simulink model "sampleModel1951"  (R2023a)
settings: Solver=VariableStepAuto  StartTime=0.0  StopTime=10.0  RelTol=1e-3
libraries: hdlsllib x3
settings Model: Creator=user1  LastModifiedBy=user1

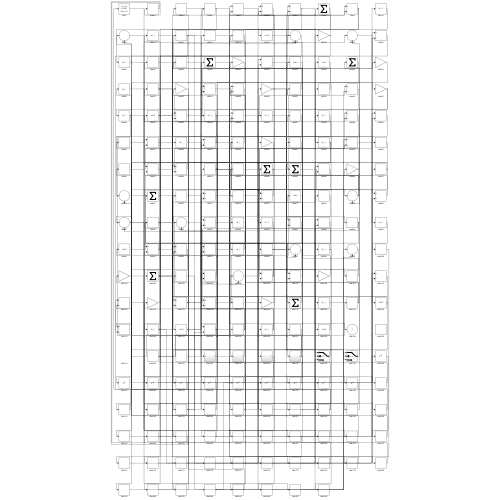
[thumbnail: Simulink's stored preview of the top-level diagram]
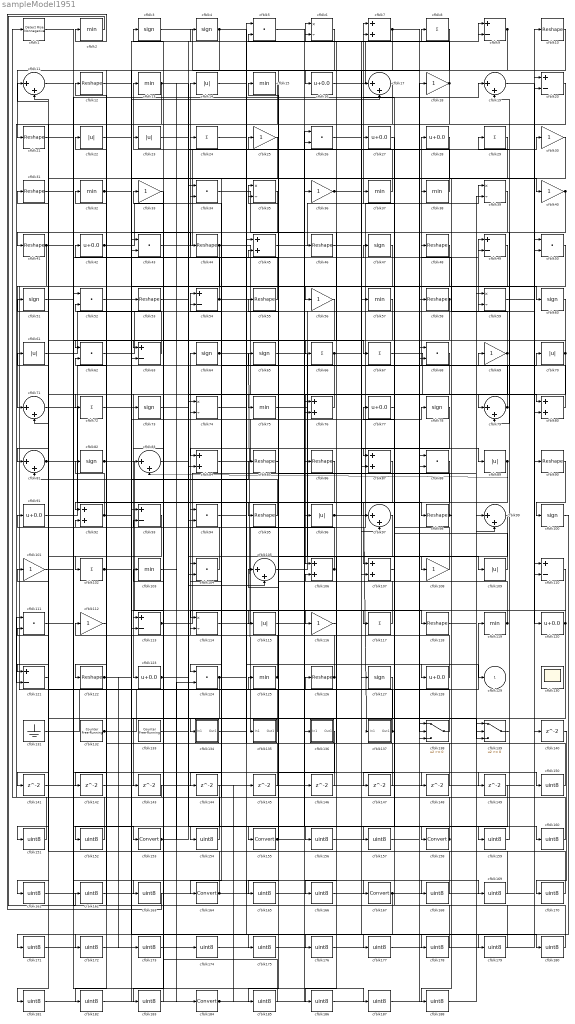
== system sampleModel1951 ==
  cfblk1 : hdlsllib/Logic and Bit Operations/Detect Rise Nonnegative  vinit=0  OutDataTypeStr=boolean
  cfblk{10,12,21,31,41,44,46,48,53,55,58,85..86,90,95,98,118,122,126} (19 alike) : Reshape
  cfblk{3..4,47,51,60,64..65,73,78,82,100,127} (12 alike) : Signum
  cfblk{18,25,30,33,36,40,56,69,101,108,112,116} (12 alike) : Gain
  cfblk{8,24,29,66..67,72,102,117} (8 alike) : Sum  Inputs=+
  cfblk{2,13,15,32,37..38,57,75,103,119,125} (11 alike) : MinMax
  cfblk{5,26,34,43,50,52,62,68,88,94,104,111,124} (13 alike) : DotProduct  OutDataTypeStr=Inherit: Inherit via internal rule
  cfblk{11,17,19,71,79,81,83,97,99,105} (10 alike) : Sum  Inputs=|++
  cfblk{7,45,76,80,84,87,92,106..107} (9 alike) : Sum
  cfblk{14,22..23,61,70,89,96,109,115} (9 alike) : Abs  SaturateOnIntegerOverflow=off
  cfblk{9,20,49,54,63,93,110,113,121} (9 alike) : Sum  Inputs=+-
  cfblk{6,35,39,59,74,114} (6 alike) : Product  Inputs=*/  RndMeth=Zero  SaturateOnIntegerOverflow=on
  cfblk{16,27..28,42,77,91,120,123,128} (9 alike) : Bias  Bias=0.0  SaturateOnIntegerOverflow=off
  cfblk130 : Scope
      settings: Floating=on
  cfblk131 : Ground
  cfblk132 : hdlsllib/Sources/Counter Free-Running  NumBits=16  tsamp=-1
  cfblk133 : hdlsllib/Sources/Counter Free-Running  NumBits=16  tsamp=-1
  cfblk134 : Subsystem
      settings: LibrarySourceBlock=|
      | hdlsllib/Ports &
      | Subsystems/Subsystem
  cfblk135 : Subsystem
      settings: LibrarySourceBlock=|
      | hdlsllib/Ports &
      | Subsystems/Subsystem
  cfblk136 : Subsystem
      settings: LibrarySourceBlock=|
      | hdlsllib/Ports &
      | Subsystems/Subsystem
  cfblk137 : Subsystem
      settings: LibrarySourceBlock=|
      | hdlsllib/Ports &
      | Subsystems/Subsystem
  cfblk138 : Switch  SaturateOnIntegerOverflow=off  InputSameDT=off
  cfblk139 : Switch  SaturateOnIntegerOverflow=off  InputSameDT=off
  cfblk{140..149} (10 alike) : Delay  SampleTime=1
  cfblk{150..152,154,156..157,159..163,165..166,168..183,185..188} (33 alike) : DataTypeConversion  OutDataTypeStr=uint8  SaturateOnIntegerOverflow=off  RndMeth=Floor
  cfblk{153,155,158,164,167,184} (6 alike) : DataTypeConversion  SaturateOnIntegerOverflow=off  RndMeth=Floor
  cfblk129 : Outport  VectorParamsAs1DForOutWhenUnconnected=off
  wires:
  cfblk29/1 -> cfblk158/1
  cfblk37/1 -> cfblk13/1
  cfblk125/1 -> cfblk64/1, cfblk62/2, cfblk45/2
  cfblk42/1 -> cfblk14/1, cfblk139/2
  cfblk41/1 -> cfblk119/1, cfblk49/2
  cfblk66/1 -> cfblk123/1, cfblk89/1
  cfblk55/1 -> cfblk24/1
  cfblk48/1 -> cfblk56/1
  cfblk70/1 -> cfblk63/1, cfblk161/1
  cfblk64/1 -> cfblk135/1(In1), cfblk138/1, cfblk180/1
  cfblk13/1 -> cfblk108/1, cfblk121/2, cfblk174/1
  cfblk71/1 -> cfblk98/1
  cfblk79/1 -> cfblk28/1, cfblk65/1
  cfblk36/1 -> cfblk139/3, cfblk179/1
  cfblk96/1 -> cfblk137/1(In1), cfblk138/2, cfblk9/2
  cfblk25/1 -> cfblk134/1(In1)
  cfblk124/1 -> cfblk7/2, cfblk151/1
  cfblk137/1(Out1) -> cfblk126/1, cfblk114/2, cfblk157/1
  cfblk10/1 -> cfblk21/1
  cfblk82/1 -> cfblk118/1, cfblk4/1
  cfblk91/1 -> cfblk69/1
  cfblk49/1 -> cfblk71/1
  cfblk87/1 -> cfblk107/1
  cfblk76/1 -> cfblk75/1
  cfblk105/1 -> cfblk20/1
  cfblk43/1 -> cfblk10/1
  cfblk9/1 -> cfblk95/1, cfblk113/2
  cfblk86/1 -> cfblk92/1
  cfblk114/1 -> cfblk39/1
  cfblk138/1 -> cfblk77/1
  cfblk28/1 -> cfblk71/2
  cfblk69/1 -> cfblk87/1, cfblk48/1
  cfblk121/1 -> cfblk51/1
  cfblk65/1 -> cfblk109/1
  cfblk50/1 -> cfblk164/1
  cfblk63/1 -> cfblk12/1
  cfblk131/1 -> cfblk45/1
  cfblk44/1 -> cfblk106/1, cfblk72/1
  cfblk16/1 -> cfblk9/1
  cfblk30/1 -> cfblk124/1
  cfblk132/1 -> cfblk125/1, cfblk94/2
  cfblk104/1 -> cfblk42/1
  cfblk8/1 -> cfblk107/2
  cfblk45/1 -> cfblk7/1
  cfblk98/1 -> cfblk35/1, cfblk188/1
  cfblk107/1 -> cfblk27/1
  cfblk75/1 -> cfblk49/1
  cfblk20/1 -> cfblk122/1
  cfblk85/1 -> cfblk115/1
  cfblk60/1 -> cfblk83/1
  cfblk118/1 -> cfblk70/1
  cfblk120/1 -> cfblk114/1, cfblk143/1
  cfblk27/1 -> cfblk117/1
  cfblk38/1 -> cfblk25/1
  cfblk59/1 -> cfblk120/1
  cfblk68/1 -> cfblk155/1
  cfblk108/1 -> cfblk23/1
  cfblk47/1 -> cfblk113/1
  cfblk128/1 -> cfblk3/1
  cfblk116/1 -> cfblk6/1
  cfblk133/1 -> cfblk30/1
  cfblk39/1 -> cfblk121/1
  cfblk51/1 -> cfblk19/1
  cfblk11/1 -> cfblk167/1
  cfblk80/1 -> cfblk54/1
  cfblk7/1 -> cfblk16/1, cfblk129/1
  cfblk112/1 -> cfblk32/1
  cfblk5/1 -> cfblk86/1
  cfblk34/1 -> cfblk136/1(In1)
  cfblk12/1 -> cfblk60/1
  cfblk67/1 -> cfblk80/1
  cfblk126/1 -> cfblk15/1, cfblk104/1
  cfblk24/1 -> cfblk97/1
  cfblk81/1 -> cfblk97/2, cfblk168/1
  cfblk94/1 -> cfblk96/1
  cfblk89/1 -> cfblk83/2, cfblk104/2
  cfblk32/1 -> cfblk53/1, cfblk44/1
  cfblk4/1 -> cfblk63/2, cfblk177/1
  cfblk109/1 -> cfblk17/1
  cfblk117/1 -> cfblk6/2
  cfblk14/1 -> cfblk128/1
  cfblk23/1 -> cfblk76/1
  cfblk53/1 -> cfblk105/2
  cfblk15/1 -> cfblk41/1
  cfblk61/1 -> cfblk34/1
  cfblk35/1 -> cfblk84/1
  cfblk1/1 -> cfblk67/1
  cfblk31/1 -> cfblk153/1
  cfblk113/1 -> cfblk59/1, cfblk8/1
  cfblk84/1 -> cfblk57/1
  cfblk139/1 -> cfblk19/2
  cfblk106/1 -> cfblk94/1, cfblk35/2
  cfblk62/1 -> cfblk38/1
  cfblk119/1 -> cfblk91/1, cfblk55/1
  cfblk92/1 -> cfblk85/1, cfblk82/1
  cfblk58/1 -> cfblk81/1, cfblk102/1
  cfblk26/1 -> cfblk79/1
  cfblk135/1(Out1) -> cfblk101/1
  cfblk103/1 -> cfblk184/1
  cfblk40/1 -> cfblk79/2, cfblk66/1
  cfblk90/1 -> cfblk100/1
  cfblk102/1 -> cfblk47/1, cfblk17/2, cfblk116/1
  cfblk95/1 -> cfblk81/2
  cfblk54/1 -> cfblk87/2, cfblk22/1
  cfblk19/1 -> cfblk90/1
  cfblk46/1 -> cfblk127/1
  cfblk18/1 -> cfblk43/2, cfblk5/2
  cfblk123/1 -> cfblk74/1, cfblk78/1
  cfblk74/1 -> cfblk59/2
  cfblk22/1 -> cfblk40/1
  cfblk3/1 -> cfblk58/1
  cfblk122/1 -> cfblk74/2, cfblk173/1
  cfblk6/1 -> cfblk62/1
  cfblk57/1 -> cfblk141/1
  cfblk141/1 -> cfblk80/2
  cfblk17/1 -> cfblk142/1
  cfblk142/1 -> cfblk20/2
  cfblk143/1 -> cfblk1/1
  cfblk56/1 -> cfblk144/1
  cfblk145/1 -> cfblk5/1
  cfblk146/1 -> cfblk92/2
  cfblk77/1 -> cfblk147/1
  cfblk147/1 -> cfblk106/2
  cfblk72/1 -> cfblk148/1
  cfblk148/1 -> cfblk54/2
  cfblk83/1 -> cfblk149/1
  cfblk111/1 -> cfblk150/1
  cfblk150/1 -> cfblk33/1
  cfblk151/1 -> cfblk111/1
  cfblk144/1 -> cfblk152/1
  cfblk152/1 -> cfblk111/2
  cfblk153/1 -> cfblk84/2, cfblk124/2
  cfblk78/1 -> cfblk154/1
  cfblk154/1 -> cfblk31/1
  cfblk155/1 -> cfblk76/2, cfblk105/1
  cfblk134/1(Out1) -> cfblk156/1
  cfblk156/1 -> cfblk68/1
  cfblk157/1 -> cfblk68/2
  cfblk158/1 -> cfblk61/1, cfblk112/1
  cfblk115/1 -> cfblk159/1
  cfblk159/1 -> cfblk29/1
  cfblk73/1 -> cfblk160/1
  cfblk160/1 -> cfblk34/2
  cfblk161/1 -> cfblk73/1
  cfblk2/1 -> cfblk162/1
  cfblk162/1 -> cfblk46/1
  cfblk101/1 -> cfblk163/1
  cfblk163/1 -> cfblk2/1
  cfblk164/1 -> cfblk43/1, cfblk169/1
  cfblk136/1(Out1) -> cfblk165/1
  cfblk165/1 -> cfblk50/1
  cfblk127/1 -> cfblk166/1
  cfblk166/1 -> cfblk50/2
  cfblk167/1 -> cfblk138/3, cfblk176/1
  cfblk168/1 -> cfblk11/1
  cfblk169/1 -> cfblk11/2
  cfblk140/1 -> cfblk170/1
  cfblk170/1 -> cfblk26/1
  cfblk100/1 -> cfblk171/1
  cfblk171/1 -> cfblk140/1
  cfblk88/1 -> cfblk172/1
  cfblk172/1 -> cfblk26/2
  cfblk173/1 -> cfblk88/1
  cfblk174/1 -> cfblk88/2
  cfblk110/1 -> cfblk175/1
  cfblk175/1 -> cfblk36/1
  cfblk176/1 -> cfblk110/1
  cfblk177/1 -> cfblk110/2
  cfblk52/1 -> cfblk178/1
  cfblk178/1 -> cfblk37/1
  cfblk179/1 -> cfblk52/1
  cfblk180/1 -> cfblk52/2
  cfblk93/1 -> cfblk181/1
  cfblk181/1 -> cfblk18/1
  cfblk149/1 -> cfblk182/1
  cfblk182/1 -> cfblk93/1
  cfblk33/1 -> cfblk183/1
  cfblk183/1 -> cfblk93/2
  cfblk184/1 -> cfblk146/1, cfblk145/1, cfblk39/2
  cfblk97/1 -> cfblk185/1
  cfblk185/1 -> cfblk103/1
  cfblk99/1 -> cfblk186/1
  cfblk186/1 -> cfblk139/1
  cfblk21/1 -> cfblk187/1
  cfblk187/1 -> cfblk99/1
  cfblk188/1 -> cfblk99/2

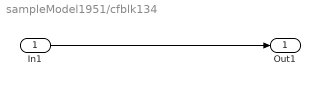
== system sampleModel1951/cfblk134 ==
  In1 : Inport
  Out1 : Outport
  wires:
  In1/1 -> Out1/1

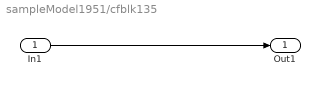
== system sampleModel1951/cfblk135 ==
  In1 : Inport
  Out1 : Outport
  wires:
  In1/1 -> Out1/1

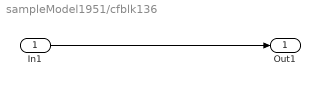
== system sampleModel1951/cfblk136 ==
  In1 : Inport
  Out1 : Outport
  wires:
  In1/1 -> Out1/1

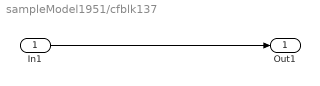
== system sampleModel1951/cfblk137 ==
  In1 : Inport
  Out1 : Outport
  wires:
  In1/1 -> Out1/1
